simulink model "PID_miniHopper_3_Pitch_Roll_Yaw_Contour_3"  (R2022b)
settings: Solver=VariableStepAuto  StartTime=0.0  StopTime=10  RelTol=1e-3
values from neighbouring files (symbols this model uses):
  hopper_ode = struct()    [MiniHopperParameters.m]
undefined symbols (not defined in the file or in its folder): A_rpy, B_rpy, Gain_pitch_U, Gain_roll_U, Gain_yaw_U, VxLoop, VyLoop, XIC_rpy, XLoop, YLoop
libraries: simulink_extras x18, slpidlib x10
(part 2 of 2)

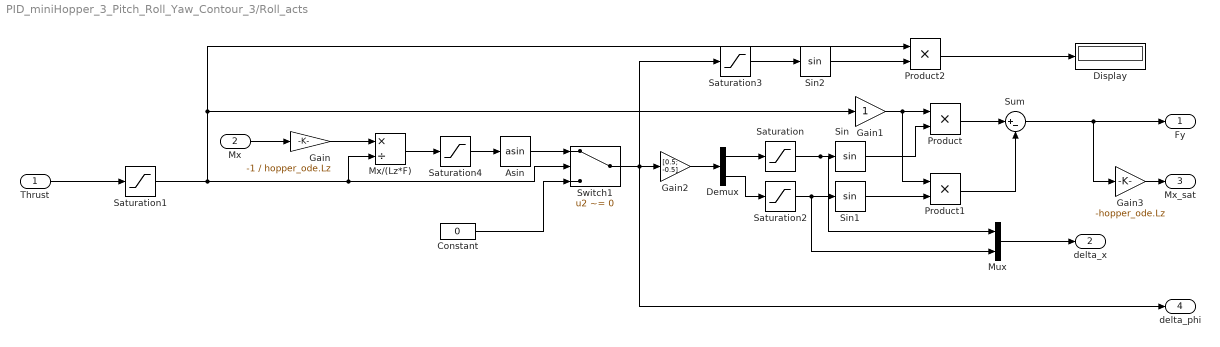
== system PID_miniHopper_3_Pitch_Roll_Yaw_Contour_3/Roll_acts ==
  Thrust : Inport
  Mx : Inport  Port=2
  Asin : Trigonometry  Operator=asin
  Constant : Constant  Value=0
  Demux : Demux  Outputs=2
  Display : Display
  Gain : Gain  Gain=-1 / hopper_ode.Lz
  Gain1 : Gain
  Gain2 : Gain  Gain=[0.5; -0.5]
  Gain3 : Gain  Gain=-hopper_ode.Lz
  Mux : Mux  Inputs=2
  Mx/(Lz*F) : Product  Inputs=*/
  Product : Product
  Product1 : Product
  Product2 : Product
  Saturation : Saturate  UpperLimit=deg2rad(45)  LowerLimit=-deg2rad(45)
  Saturation1 : Saturate  UpperLimit=25  LowerLimit=0
  Saturation2 : Saturate  UpperLimit=deg2rad(45)  LowerLimit=-deg2rad(45)
  Saturation3 : Saturate  UpperLimit=deg2rad(45)  LowerLimit=-deg2rad(45)
  Saturation4 : Saturate  UpperLimit=1  LowerLimit=-1
  Sin : Trigonometry
  Sin1 : Trigonometry
  Sin2 : Trigonometry
  Sum : Sum  Inputs=|+-
  Switch1 : Switch  Criteria=u2 ~= 0  SaturateOnIntegerOverflow=off  InputSameDT=off
  Fy : Outport
  delta_x : Outport  Port=2
  Mx_sat : Outport  Port=3
  delta_phi : Outport  Port=4
  wires:
  Saturation4/1 -> Asin/1
  Gain3/1 -> Mx_sat/1
  Asin/1 -> Switch1/1
  Gain1/1 -> Product/1, Product1/1
  Product2/1 -> Display/1
  Saturation1/1 -> Product2/1, Gain1/1, Mx/(Lz*F)/2, Switch1/2
  Sin2/1 -> Product2/2
  Saturation3/1 -> Sin2/1
  Product1/1 -> Sum/2
  Sum/1 -> Fy/1, Gain3/1
  Sin1/1 -> Product1/2
  Mux/1 -> delta_x/1
  Saturation2/1 -> Sin1/1, Mux/2
  Demux/2 -> Saturation2/1
  Demux/1 -> Saturation/1
  Gain2/1 -> Demux/1
  Saturation/1 -> Sin/1, Mux/1
  Thrust/1 -> Saturation1/1
  Constant/1 -> Switch1/3
  Switch1/1 -> delta_phi/1, Gain2/1, Saturation3/1
  Product/1 -> Sum/1
  Sin/1 -> Product/2
  Mx/(Lz*F)/1 -> Saturation4/1
  Gain/1 -> Mx/(Lz*F)/1
  Mx/1 -> Gain/1

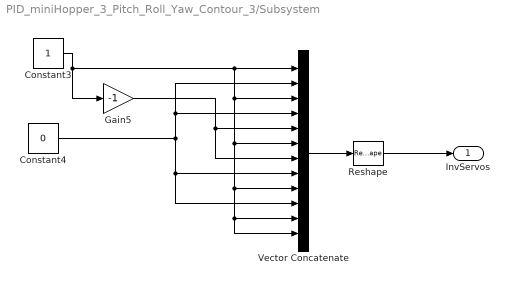
== system PID_miniHopper_3_Pitch_Roll_Yaw_Contour_3/Subsystem ==
  Constant3 : Constant
  Constant4 : Constant  Value=0
  Gain5 : Gain  Gain=-1
  Reshape : Reshape  OutputDimensionality=Customize  OutputDimensions=[3,4]
  Vector Concatenate : Concatenate  NumInputs=12
  InvServos : Outport
  wires:
  Constant3/1 -> Vector Concatenate/1, Vector Concatenate/12, Vector Concatenate/11, Vector Concatenate/9, Vector Concatenate/6, Vector Concatenate/3, Gain5/1
  Constant4/1 -> Vector Concatenate/2, Vector Concatenate/4, Vector Concatenate/10, Vector Concatenate/8
  Vector Concatenate/1 -> Reshape/1
  Gain5/1 -> Vector Concatenate/7, Vector Concatenate/5
  Reshape/1 -> InvServos/1

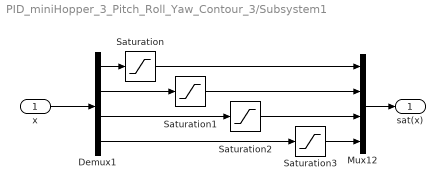
== system PID_miniHopper_3_Pitch_Roll_Yaw_Contour_3/Subsystem1 ==
  x : Inport
  Demux1 : Demux
  Mux12 : Mux
  Saturation{,1..3} (4 alike) : Saturate  UpperLimit=deg2rad(45)  LowerLimit=-deg2rad(45)
  sat(x) : Outport
  wires:
  Demux1/3 -> Saturation2/1
  Demux1/4 -> Saturation3/1
  Demux1/1 -> Saturation/1
  Demux1/2 -> Saturation1/1
  x/1 -> Demux1/1
  Mux12/1 -> sat(x)/1
  Saturation/1 -> Mux12/1
  Saturation1/1 -> Mux12/2
  Saturation2/1 -> Mux12/3
  Saturation3/1 -> Mux12/4

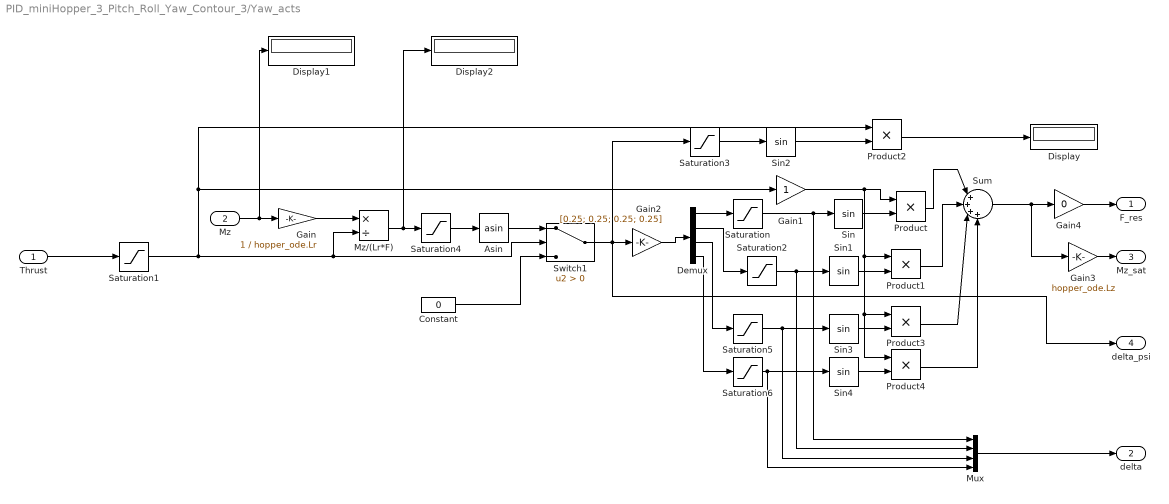
== system PID_miniHopper_3_Pitch_Roll_Yaw_Contour_3/Yaw_acts ==
  Thrust : Inport
  Mz : Inport  Port=2
  Asin : Trigonometry  Operator=asin
  Constant : Constant  Value=0
  Demux : Demux
  Display : Display
  Display1 : Display
  Display2 : Display
  Gain : Gain  Gain=1 / hopper_ode.Lr
  Gain1 : Gain
  Gain2 : Gain  Gain=[0.25; 0.25; 0.25; 0.25]
  Gain3 : Gain  Gain=hopper_ode.Lz
  Gain4 : Gain  Gain=0
  Mux : Mux
  Mz/(Lr*F) : Product  Inputs=*/
  Product{,1..4} (5 alike) : Product
  Saturation{,2..3,5..6} (5 alike) : Saturate  UpperLimit=deg2rad(45)  LowerLimit=-deg2rad(45)
  Saturation1 : Saturate  UpperLimit=25  LowerLimit=0
  Saturation4 : Saturate  UpperLimit=1  LowerLimit=-1
  Sin{,1..4} (5 alike) : Trigonometry
  Sum : Sum  Inputs=|++++
  Switch1 : Switch  Criteria=u2 > Threshold  SaturateOnIntegerOverflow=off  InputSameDT=off
  F_res : Outport
  delta : Outport  Port=2
  Mz_sat : Outport  Port=3
  delta_psi : Outport  Port=4
  wires:
  Mz/1 -> Display1/1, Gain/1
  Gain/1 -> Mz/(Lr*F)/1
  Mz/(Lr*F)/1 -> Display2/1, Saturation4/1
  Sin/1 -> Product/2
  Product/1 -> Sum/1
  Switch1/1 -> delta_psi/1, Saturation3/1, Gain2/1
  Constant/1 -> Switch1/3
  Thrust/1 -> Saturation1/1
  Saturation/1 -> Sin/1, Mux/1
  Gain2/1 -> Demux/1
  Demux/1 -> Saturation/1
  Demux/2 -> Saturation2/1
  Saturation2/1 -> Mux/2, Sin1/1
  Mux/1 -> delta/1
  Sin1/1 -> Product1/2
  Sum/1 -> Gain4/1, Gain3/1
  Product1/1 -> Sum/2
  Saturation3/1 -> Sin2/1
  Sin2/1 -> Product2/2
  Saturation1/1 -> Switch1/2, Mz/(Lr*F)/2, Gain1/1, Product2/1
  Product2/1 -> Display/1
  Gain1/1 -> Product1/1, Product4/1, Product3/1, Product/1
  Asin/1 -> Switch1/1
  Gain3/1 -> Mz_sat/1
  Saturation4/1 -> Asin/1
  Demux/3 -> Saturation5/1
  Saturation5/1 -> Sin3/1, Mux/3
  Saturation6/1 -> Sin4/1, Mux/4
  Sin3/1 -> Product3/2
  Sin4/1 -> Product4/2
  Product3/1 -> Sum/3
  Product4/1 -> Sum/4
  Demux/4 -> Saturation6/1
  Gain4/1 -> F_res/1

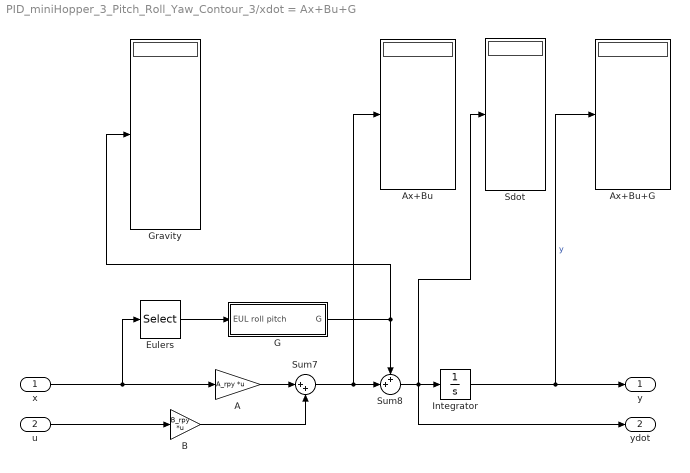
== system PID_miniHopper_3_Pitch_Roll_Yaw_Contour_3/xdot = Ax+Bu+G ==
  x : Inport
  u : Inport  Port=2
  A : Gain  Gain=A_rpy  Multiplication=Matrix(K*u)
  Ax+Bu : Display
  Ax+Bu+G : Display
  B : Gain  Gain=B_rpy  Multiplication=Matrix(K*u)
  Eulers : Selector  InputPortWidth=10  IndexOptions=Index vector (dialog)  Indices=[5 6 7]  OutputSizes=1
  G : Subsystem
  Gravity : Display
  Integrator : Integrator  InitialCondition=XIC_rpy
  Sdot : Display
  Sum7 : Sum  Inputs=|++
  Sum8 : Sum  Inputs=++|
  y : Outport
  ydot : Outport  Port=2
  wires:
  u/1 -> B/1
  B/1 -> Sum7/2
  Sum7/1 -> Ax+Bu/1, Sum8/2
  A/1 -> Sum7/1
  G/1(G) -> Gravity/1, Sum8/1
  x/1 -> Eulers/1, A/1
  Integrator/1 -> Ax+Bu+G/1, y/1  "y"
  Eulers/1 -> G/1(EUL roll pitch)
  Sum8/1 -> Sdot/1, ydot/1, Integrator/1

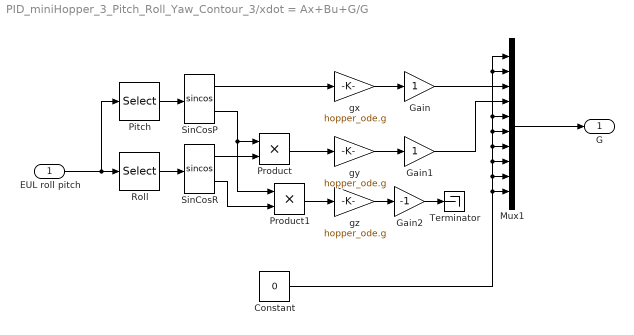
== system PID_miniHopper_3_Pitch_Roll_Yaw_Contour_3/xdot = Ax+Bu+G/G ==
  EUL roll pitch : Inport
  Constant : Constant  Value=0
  Gain : Gain
  Gain1 : Gain
  Gain2 : Gain  Gain=-1
  Mux1 : Mux  Inputs=10
  Pitch : Selector  InputPortWidth=3  IndexOptions=Index vector (dialog)  Indices=[2]  OutputSizes=1
  Product : Product
  Product1 : Product
  Roll : Selector  InputPortWidth=3  IndexOptions=Index vector (dialog)  Indices=[1]  OutputSizes=1
  SinCosP : Trigonometry  Operator=sincos
  SinCosR : Trigonometry  Operator=sincos
  Terminator : Terminator
  gx : Gain  Gain=hopper_ode.g
  gy : Gain  Gain=hopper_ode.g
  gz : Gain  Gain=hopper_ode.g
  G : Outport
  wires:
  Gain/1 -> Mux1/3
  Mux1/1 -> G/1
  Roll/1 -> SinCosR/1
  EUL roll pitch/1 -> Pitch/1, Roll/1
  SinCosP/2 -> Product1/1, Product/1
  SinCosR/1 -> Product/2
  gx/1 -> Gain/1
  Pitch/1 -> SinCosP/1
  SinCosP/1 -> gx/1
  Product/1 -> gy/1
  gy/1 -> Gain1/1
  Gain1/1 -> Mux1/4
  SinCosR/2 -> Product1/2
  Product1/1 -> gz/1
  gz/1 -> Gain2/1
  Gain2/1 -> Terminator/1
  Constant/1 -> Mux1/2, Mux1/1, Mux1/5, Mux1/6, Mux1/7, Mux1/8, Mux1/9, Mux1/10
